simulink model "pendulo"  (R2015a)
settings: Solver=ode45  StartTime=0.0  StopTime=10.0  MaxStep=0.01  MinStep=0.001  RelTol=1e-3
values from neighbouring files (symbols this model uses):
  p10 = 0    [lab1.m]
  p20 = 0    [lab1.m]
  t10 = teta10(i)    [lab1.m]
  t20 = teta20(i)    [lab1.m]
settings Model: Creator=João F  LastModifiedBy=João F
settings DebuggingCC: UnderspecifiedInitializationDetection=Classic  MergeDetectMultiDrivingBlocksExec=none  SolverPrmCheckMsg=warning  StateNameClashWarn=warning

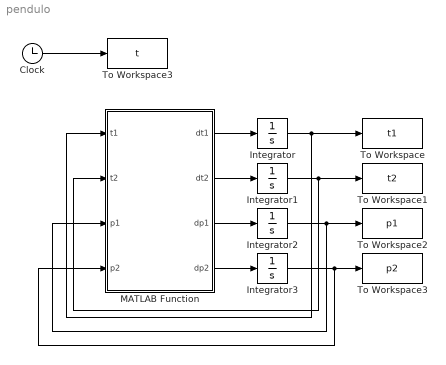
== system pendulo ==
  Clock : Clock
  Integrator : Integrator  InitialCondition=t10
  Integrator1 : Integrator  InitialCondition=t20
  Integrator2 : Integrator  InitialCondition=p10
  Integrator3 : Integrator  InitialCondition=p20
  MATLAB Function : MATLAB Function  TreatAsAtomicUnit=on
      settings: PermitHierarchicalResolution=ParametersOnly
  To Workspace : ToWorkspace  VariableName=t1  SampleTime=-1
  To Workspace1 : ToWorkspace  VariableName=t2  SampleTime=-1
  To Workspace2 : ToWorkspace  VariableName=p1  SampleTime=-1
  To Workspace3 : ToWorkspace  VariableName=p2  SampleTime=-1
  "To Workspace3 " : ToWorkspace  VariableName=t  SampleTime=-1
  wires:
  Clock/1 -> "To Workspace3 "/1
  MATLAB Function/1(dt1) -> Integrator/1
  Integrator/1 -> To Workspace/1, MATLAB Function/1(t1)
  Integrator2/1 -> MATLAB Function/3(p1), To Workspace2/1
  Integrator3/1 -> MATLAB Function/4(p2), To Workspace3/1
  Integrator1/1 -> MATLAB Function/2(t2), To Workspace1/1
  MATLAB Function/2(dt2) -> Integrator1/1
  MATLAB Function/3(dp1) -> Integrator2/1
  MATLAB Function/4(dp2) -> Integrator3/1

== matlab function pendulo/MATLAB Function ==
  data: t1 input; dt1 output; t2 input; p1 input; p2 input; dt2 output; dp1 output; dp2 output
function [dt1,dt2,dp1,dp2] = pendulo(t1,t2,p1,p2)

%Aceleração Gravítica, massa e comprimento do pêndulo.
g=9.8;
m=1;
l=0.5;

%Derivada de Teta1
dt1=(6/(m*l^2))*(2*p1-3*cos(t1-t2)*p2)/(16-9*cos(t1-t2)^2);

%Derivada de Teta2
dt2=(6/(m*l^2))*(8*p2-3*cos(t1-t2)*p1)/(16-9*cos(t1-t2)^2);

%Derivada da Velocidade Ângular 1
dp1=((-1/2)*m*l^2)*(dt1*dt2*sin(t1-t2)+3*(g/l)*sin(t1));

%Derivada da Velocidade Ângular 2
dp2=((-1/2)*m*l^2)*(-dt1*dt2*sin(t1-t2)+(g/l)*sin(t2));
